simulink model "DCMotorControlSystem"  (R2013a)
settings: Solver=ode45  StartTime=0.0  StopTime=0.5  MaxStep=1e-6  RelTol=1e-4
values from neighbouring files (symbols this model uses):
  b = kps - B    (= 0.314159265359)    [Script_IMC.m]
  J = 1e-3    (= 0.001)    [Script_IMC.m]
  kf = 0.35    [Script_IMC.m]
  kic = alphac^2*La    (= 24674.0110027)    [Script_IMC.m]
  kis = (alphas^2)*J    (= 98.6960440109)    [Script_IMC.m]
  kpc = alphac*La    (= 7.85398163397)    [Script_IMC.m]
  kps = alphas*J    (= 0.314159265359)    [Script_IMC.m]
  La = 2.5e-3    (= 0.0025)    [Script_IMC.m]
  r = kpc - Ra    (= 7.35398163397)    [Script_IMC.m]
  Ra = 0.5    [Script_IMC.m]
  Tmax = 2*TN    (= 14)    [Script_IMC.m]
  Tmin = -2*TN    (= -14)    [Script_IMC.m]
  Tsw = 1e-4    (= 0.0001)    [Script_IMC.m]
  Udc = 140    [Script_IMC.m]
  Umax = 140    [Script_IMC.m]
  Umin = -140    [Script_IMC.m]
libraries: powerlib x8, simulink x1, powerlib_meascontrol x1
settings Model: Creator=osinowo paul  LastModifiedBy=osinowo paul
settings SolverCC: ZeroCrossAlgorithm=Adaptive
settings DebuggingCC: MaskedZcDiagnostic=none

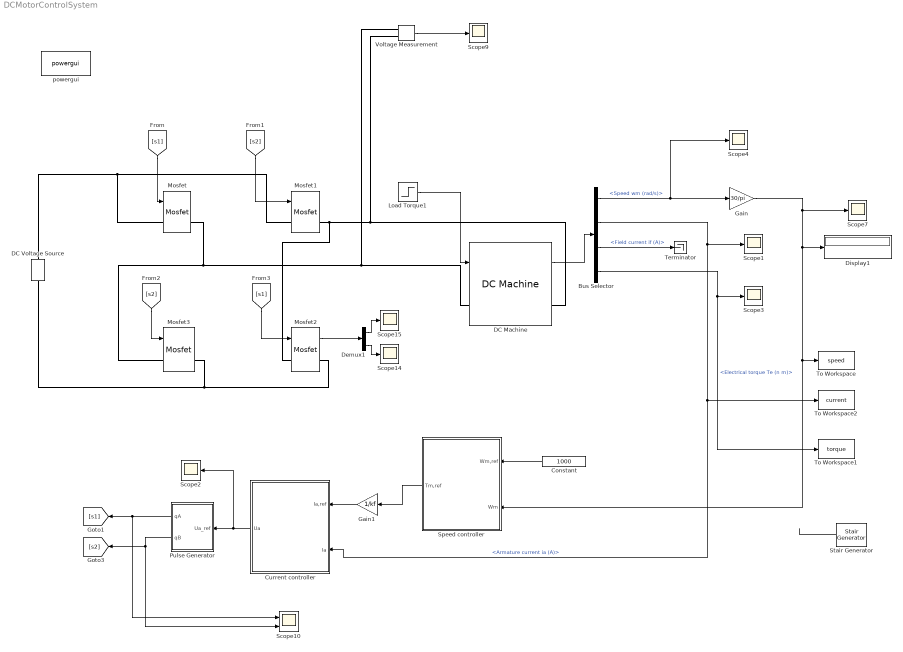
== system DCMotorControlSystem ==
  Bus Selector : BusSelector  OutputSignals=Speed wm (rad/s),Armature current ia (A),Field current if (A),Electrical torque Te (n m)
  Constant : Constant  Value=1000
  Current controller : Subsystem
  DC Machine : powerlib/Machines/DC Machine  PresetModel=No  MechanicalLoad=Torque TL  FieldType=Permanent magnet  ShowDetailedParameters=on  RLa="[Ra  La]"  RLf="[ 240  120]"  Laf=1.8  MachineConstant=Torque constant (N.m/A)  Ke=1.8  Kt=kf  J=J  Bm=0  Tf=0  w0=0  Ifinit=1  TsPowergui=0  TsBlock=-1
  DC Voltage Source : powerlib/Electrical Sources/DC Voltage Source  Amplitude=Udc  Measurements=None
  Demux1 : Demux  Outputs=2
  Display1 : Display
  Gain : Gain  Gain=30/pi
  Gain1 : Gain  Gain=1/kf
  Load Torque1 : Step  Time=0.04  After=0.2  SampleTime=0
  Mosfet{,1..3} (4 alike) : powerlib/Power Electronics/Mosfet  Ron=0.1  Lon=0  Rd=0.01  Vfd=0  IC=0  Rs=1e5  Cs=inf  Measurements=on
  Pulse Generator : Subsystem
  Scope{1..4,7,9,14..15} (8 alike) : Scope
      Scope1 settings: TimeRange=0.5  YMin=12.9019  YMax=12.9022  SaveName=ScopeData6
      Scope14 settings: TimeRange=2  YMin=-150  YMax=150  SaveName=ScopeData15
      Scope15 settings: TimeRange=2  YMin=-150  YMax=150  SaveName=ScopeData16
      Scope2 settings: TimeRange=2  YMin=-150  YMax=150  SaveName=ScopeData7
      Scope3 settings: TimeRange=10  YMin=-2  YMax=2  SaveName=ScopeData8
      Scope4 settings: YMin=99.484  YMax=109.956
      Scope7 settings: TimeRange=8.019341754342716e-06  YMin=1500.016496378698  YMax=1500.018437491124  SaveName=ScopeData3
      Scope9 settings: TimeRange=0.04015544041450775  YMin=-40  YMax=40  SaveName=ScopeData5
  Scope10 : Scope  NumInputPorts=2
      settings: TimeRange=0.03581488933601607  YMin=-2~-2  YMax=2~2  SaveName=ScopeData9
  Speed controller : Subsystem
  Stair Generator : powerlib_meascontrol/Pulse & Signal Generators/Stair Generator  t=[0, 0.1]  e=[1000, 0]  Ts=0
  Terminator : Terminator
  To Workspace : ToWorkspace  VariableName=speed  SampleTime=-1  SaveFormat=Timeseries
  To Workspace1 : ToWorkspace  VariableName=torque  SampleTime=-1  SaveFormat=Timeseries
  To Workspace2 : ToWorkspace  VariableName=current  SampleTime=-1  SaveFormat=Timeseries
  Voltage Measurement : powerlib/Measurements/Voltage Measurement  PhasorSimulation=off  OutputType=Complex  PSBequivalent=0
  powergui : powerlib/powergui  Priority=1  SimulationMode=Continuous  SolverType=Tustin  SampleTime=50e-6  frequency=60  SPID=off  DisableSnubberDevices=off  DisableRonSwitches=off  DisableVfSwitches=off  SwTol=0  Interpol=off  DisplayEquations=off  frequencyindice=0  Pbase=100e6  ErrMax=1e-4  Iterations=50  UnitsV=V  UnitsW=MW  FunctionMessages=off  echomessages=off  HookPort=off  EnableUseOfTLC=off  x0status=blocks  RestoreLinks=warning  ResistiveCurrentMeasurement=off  Frange=[0:2:500]  Ylog=off  Xlog=on  ShowGrid=off  save=off  variable=ZData  ZoomFFT=off  StartTime=0.0  cycles=1  DisplayStyle=1  fundamental=60  FreqAxis=off  MaxFrequency=1000  frequencyindicesteady=1  RmsSteady=1  display=off  Ts=0  methode=off
  wires:
  [s2] -> Mosfet3/1
  [s1] -> Mosfet2/1
  [s1] -> Mosfet/1
  [s2] -> Mosfet1/1
  DC Machine/1 -> Bus Selector/1
  Bus Selector/1 -> Scope4/1, Gain/1  "<Speed wm (rad/s)>"
  Bus Selector/2 -> Current controller/2(" Ia"), To Workspace2/1, Scope1/1  "<Armature current ia (A)>"
  Bus Selector/3 -> Terminator/1  "<Field current if (A)>"
  Bus Selector/4 -> To Workspace1/1, Scope3/1  "<Electrical torque Te (n m)>"
  Gain/1 -> To Workspace/1, Speed controller/2("  Wm"), Display1/1, Scope7/1
  ? -> ?
  Voltage Measurement/1 -> Scope9/1
  Gain1/1 -> Current controller/1(Ia,ref)
  Speed controller/1(Tm,ref) -> Gain1/1
  Pulse Generator/1("qA ") -> [s1], Scope10/1
  Pulse Generator/2(qB) -> [s2], Scope10/2
  Current controller/1(Ua) -> Scope2/1, Pulse Generator/1(Ua_ref)
  Mosfet2/1 -> Demux1/1
  Demux1/2 -> Scope14/1
  Demux1/1 -> Scope15/1
  Stair Generator/1 -> ?
  Load Torque1/1 -> DC Machine/1
  Constant/1 -> Speed controller/1(Wm,ref)
  connections:
  DC Voltage Source/RConn1 -- Mosfet1/LConn1 -- Mosfet/LConn1
  DC Voltage Source/LConn1 -- Mosfet2/RConn1 -- Mosfet3/RConn1
  Mosfet/RConn1 -- DC Machine/LConn1 -- Voltage Measurement/LConn1 -- Mosfet3/LConn1
  Mosfet1/RConn1 -- DC Machine/RConn1 -- Voltage Measurement/LConn2 -- Mosfet2/LConn1

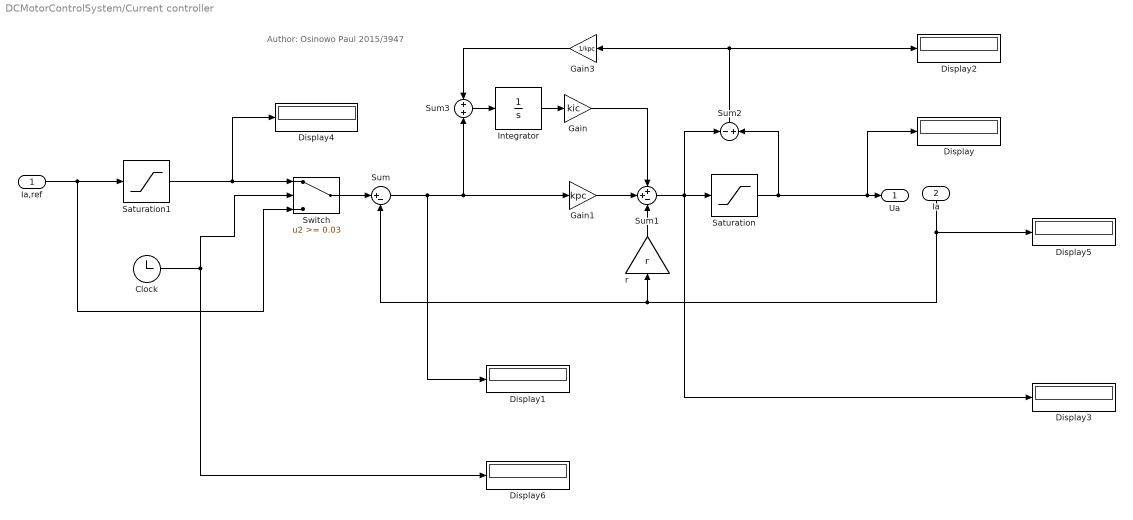
== system DCMotorControlSystem/Current controller ==
  note: Author: Osinowo Paul 2015/3947
  Ia,ref : Inport
  " Ia" : Inport  Port=2
  Clock : Clock
  Display{,1..6} (7 alike) : Display
  Gain : Gain  Gain=kic
  Gain1 : Gain  Gain=kpc
  Gain3 : Gain  Gain=1/kpc
  Integrator : Integrator
  Saturation : Saturate  UpperLimit=Umax  LowerLimit=Umin
  Saturation1 : Saturate  UpperLimit=5.4  LowerLimit=-5.4
  Sum : Sum  Inputs=|+-
  Sum1 : Sum  Inputs=++-
  Sum2 : Sum  Inputs=-|+
  Sum3 : Sum  Inputs=+|+
  Switch : Switch  Threshold=0.03
  r : Gain  Gain=r
  Ua : Outport
  wires:
  Integrator/1 -> Gain/1
  Sum1/1 -> Sum2/1, Saturation/1, Display3/1
  Gain1/1 -> Sum1/2
  Gain3/1 -> Sum3/1
  Gain/1 -> Sum1/1
  Sum/1 -> Display1/1, Gain1/1, Sum3/2
  Sum3/1 -> Integrator/1
  r/1 -> Sum1/3
  Sum2/1 -> Display2/1, Gain3/1
  " Ia"/1 -> Display5/1, Sum/2, r/1
  Saturation/1 -> Sum2/2, Display/1, Ua/1
  Ia,ref/1 -> Switch/3, Saturation1/1
  Clock/1 -> Switch/2, Display6/1
  Switch/1 -> Sum/1
  Saturation1/1 -> Display4/1, Switch/1

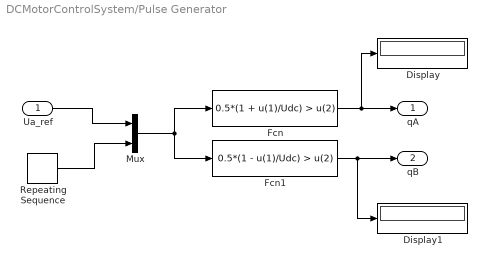
== system DCMotorControlSystem/Pulse Generator ==
  Ua_ref : Inport
  Display : Display
  Display1 : Display
  Fcn : Fcn  Expr=0.5*(1 + u(1)/Udc) > u(2)
  Fcn1 : Fcn  Expr=0.5*(1 - u(1)/Udc) > u(2)
  Mux : Mux  Inputs=2
  Repeating Sequence : simulink/Sources/Repeating Sequence  rep_seq_t=Tsw*[0 0.5 1]  rep_seq_y=[1 0 1]
  "qA " : Outport
  qB : Outport  Port=2
  wires:
  Fcn/1 -> Display/1, "qA "/1
  Repeating Sequence/1 -> Mux/2
  Fcn1/1 -> Display1/1, qB/1
  Ua_ref/1 -> Mux/1
  Mux/1 -> Fcn/1, Fcn1/1

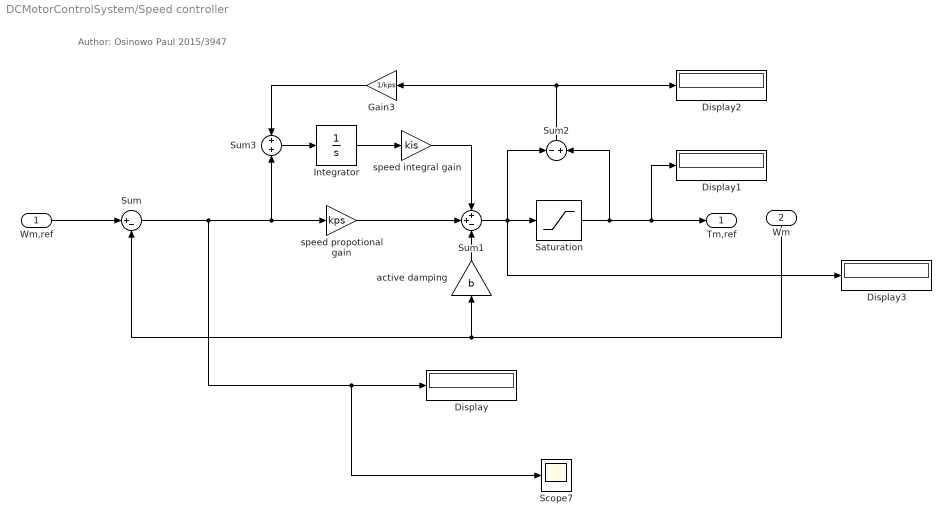
== system DCMotorControlSystem/Speed controller ==
  note: Author: Osinowo Paul 2015/3947
  Wm,ref : Inport
  "  Wm" : Inport  Port=2
  Display{,1..3} (4 alike) : Display
  Gain3 : Gain  Gain=1/kps
  Integrator : Integrator
  Saturation : Saturate  UpperLimit=Tmax  LowerLimit=Tmin
  Scope7 : Scope
      settings: TimeRange=0.5  YMin=989.5  YMax=1000.5  SaveName=ScopeData10
  Sum : Sum  Inputs=|+-
  Sum1 : Sum  Inputs=++-
  Sum2 : Sum  Inputs=-|+
  Sum3 : Sum  Inputs=+|+
  active damping : Gain  Gain=b
  speed integral gain : Gain  Gain=kis
  speed propotional gain : Gain  Gain=kps
  Tm,ref : Outport
  wires:
  "  Wm"/1 -> Sum/2, active damping/1
  Sum2/1 -> Display2/1, Gain3/1
  active damping/1 -> Sum1/3
  Sum3/1 -> Integrator/1
  Saturation/1 -> Sum2/2, Display1/1, Tm,ref/1
  speed integral gain/1 -> Sum1/1
  Gain3/1 -> Sum3/1
  Wm,ref/1 -> Sum/1
  speed propotional gain/1 -> Sum1/2
  Sum1/1 -> Sum2/1, Saturation/1, Display3/1
  Integrator/1 -> speed integral gain/1
  Sum/1 -> speed propotional gain/1, Sum3/2, Scope7/1, Display/1
